simulink model "BeamFormer"  (R2018b)
settings: Solver=VariableStepAuto  StartTime=0.0  StopTime=10.0  RelTol=1e-3
undefined symbols (not defined in the file or in its folder): phased, physconst
libraries: phasedbflib x1
settings Model: Creator=khristian  LastModifiedBy=khristian

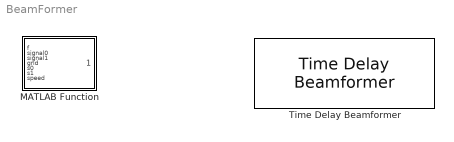
== system BeamFormer ==
  MATLAB Function : MATLAB Function  TreatAsAtomicUnit=on
  Time Delay Beamformer : phasedbflib/Time Delay Beamformer  PropagationSpeed=physconst( 'LightSpeed' )  SampleRateFromInputCheckbox=on  SampleRate=1e6  DirectionSource=Property  Direction=[ 0; 0 ]  WeightsOutputPort=off  SimulateUsing=Interpreted execution  SensorArray=phased.ULA('Element',phased.IsotropicAntennaElement)
      settings: SourceProductName=Phased Array System Toolbox  SourceProductBaseCode=AR

== matlab function BeamFormer/MATLAB Function ==
  data: f input; heatmap output; signal0 input; signal1 input; grid input; s0 input; s1 input; speed input
function heatmap  = predict(f,signal0,signal1,grid,s0,s1,speed)

    data = [];
    amp = 0;
    
    heatmap = cell(329,329);
   
  % Iterate through all grid points
    for i = 1:329
        for k = 1:329
            
            % Calculate distance from current grid point to each sensor
            distance0 = distance(s0,grid{i,k});
            distance1 = distance(s1,grid{i,k});
            
            % Determine difference in distance to reach sensor 1-3 compared
            % to reference sensor 0
            delta_1 = distance1 - distance0;

            
            % Calculate wavelength from speed of sound
            wave_length = speed/10;
            
            % Calculate phase shifts from wavelength
            shift_1 = delta_1/wave_length;

            
            % Shift signals 1-3 accordingly, in attempt to match signal 0
        

            signal1_shift = circshift(signal1,round(-shift_1.*f/10));

            % Sum all four signals
            beam1 = signal0 .*signal1_shift;

            beamformed = beam1;
            
            % Calculate root mean square ampltitude
            amplitude = mean(sqrt(beamformed.^2));
            %amplitude = max(beamformed);
            
            if amplitude > amp
                amp = amplitude;
                sig0 = signal0;
                sig1 = signal1_shift;
            end
            
            heatmap{i,k} = amplitude;
   
            data = [data amplitude];
            
        end
    end
    

end
